simulink model "diabetes_2sim"  (R2012b)
settings: Solver=ode45  StartTime=0.0  StopTime=24  RelTol=1e-3
StopFcn:
  | plot_results
libraries: simulink x2, realtime_pacer_lib x1
settings Model: Creator=tsladeche  LastModifiedBy=John
settings DataIOCC: SignalLoggingSaveFormat=ModelDataLogs
settings DebuggingCC: FcnCallInpInsideContextMsg=UseLocalSettings  StrictBusMsg=Warning
settings GRTTargetCC: CombineOutputUpdateFcns=off  GRTInterface=on

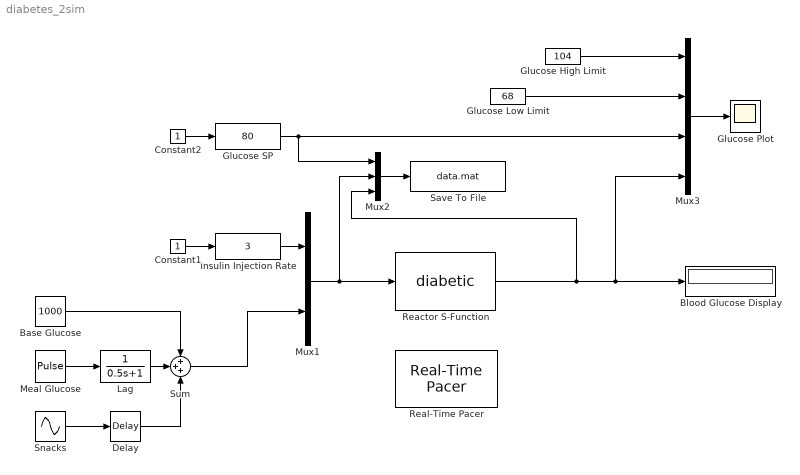
== system diabetes_2sim ==
  Base Glucose : Constant  Value=1000
  Blood Glucose Display : Display
  Constant1 : Constant
  Constant2 : Constant
  Delay : TransportDelay  DelayTime=8
  Glucose High Limit : Constant  Value=104
  Glucose Low Limit : Constant  Value=68
  Glucose Plot : Scope
      settings: ShowLegends=on  TimeRange=24  YMin=67.5  YMax=122.5  MaxDataPoints=30000
  Glucose SP : simulink/Math Operations/Slider Gain  low=50  gain=80  high=120
  Insulin Injection Rate : simulink/Math Operations/Slider Gain  low=0  gain=3  high=10
  Lag : TransferFcn  Denominator=[0.5 1]
  Meal Glucose : DiscretePulseGenerator  PulseType=Time based  Amplitude=1000  Period=6  PulseWidth=10  PhaseDelay=7
  Mux1 : Mux  Inputs=2
  Mux2 : Mux  Inputs=3
  Mux3 : Mux
  Reactor S-Function : S-Function  FunctionName=diabetic  EnableBusSupport=off
  Real-Time Pacer : realtime_pacer_lib/Real-Time Pacer  simTimePerRealTime=1
  Save To File : ToFile  Filename=data.mat  MatrixName=diabetic  SampleTime=0.05
  Snacks : Sin  Amplitude=50  SampleTime=0
  Sum : Sum  Inputs=+++
  wires:
  Mux2/1 -> Save To File/1
  Constant1/1 -> Insulin Injection Rate/1
  Mux1/1 -> Mux2/2, Reactor S-Function/1
  Constant2/1 -> Glucose SP/1
  Glucose SP/1 -> Mux3/3, Mux2/1
  Reactor S-Function/1 -> Mux3/4, Blood Glucose Display/1, Mux2/3
  Glucose High Limit/1 -> Mux3/1
  Glucose Low Limit/1 -> Mux3/2
  Mux3/1 -> Glucose Plot/1
  Insulin Injection Rate/1 -> Mux1/1
  Base Glucose/1 -> Sum/1
  Snacks/1 -> Delay/1
  Delay/1 -> Sum/3
  Meal Glucose/1 -> Lag/1
  Sum/1 -> Mux1/2
  Lag/1 -> Sum/2
